simulink subsystem "frame_ctrl"  (R2021b)
settings: Solver=VariableStepAuto  StartTime=0.0  StopTime=10.0  RelTol=1e-3
undefined symbols (not defined in the file or in its folder): bank_bitwidth, fn_bitwidth, id_bitwidth
settings Model: Creator=torha  LastModifiedBy=torha
settings SolverCC: AlgebraicLoopSolver=TrustRegion
settings DebuggingCC: SFMachineParentedDataDiag=warning

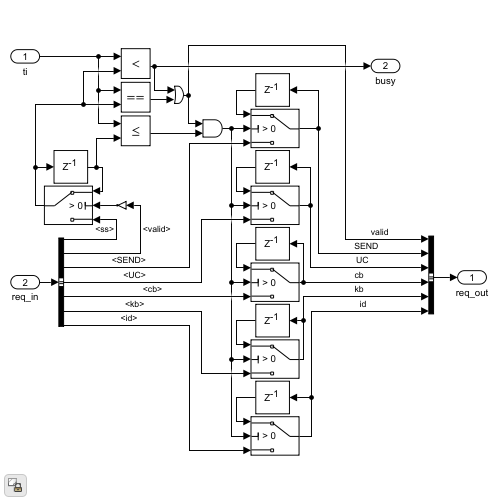
[thumbnail: Simulink's stored preview of the top-level diagram]
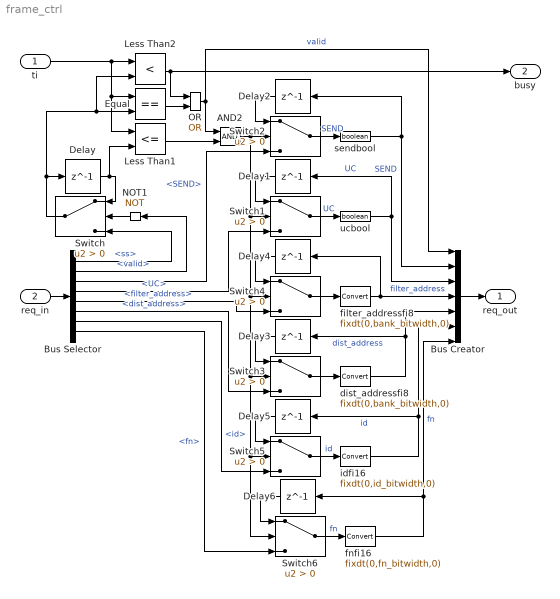
== system frame_ctrl ==
  ti : Inport
  req_in : Inport  Port=2
  AND2 : Logic  IconShape=distinctive  AllPortsSameDT=off  OutDataTypeStr=boolean
  Bus Creator : BusCreator  Inputs=7
  Bus Selector : BusSelector  OutputSignals=req.ss,valid,req.SEND,req.UC,req.filter_address,req.dist_address,id,req.fn
  Delay : Delay  DelayLength=1  InitialCondition=0
  Delay1 : Delay  DelayLength=1  InitialCondition=false
  Delay2 : Delay  DelayLength=1  InitialCondition=false
  Delay3 : Delay  DelayLength=1  InitialCondition=fi(0, false, bank_bitwidth, 0)
  Delay4 : Delay  DelayLength=1  InitialCondition=fi(0, false, bank_bitwidth, 0)
  Delay5 : Delay  DelayLength=1  InitialCondition=fi(0, false, id_bitwidth, 0)
  Delay6 : Delay  DelayLength=1  InitialCondition=fi(0, false, fn_bitwidth, 0)
  Equal : RelationalOperator  Operator===  OutDataTypeStr=boolean  RndMeth=Simplest
  Less Than1 : RelationalOperator  Operator=<=  OutDataTypeStr=boolean  RndMeth=Simplest
  Less Than2 : RelationalOperator  Operator=<  OutDataTypeStr=boolean  RndMeth=Simplest
  NOT1 : Logic  Operator=NOT  IconShape=distinctive  AllPortsSameDT=off  OutDataTypeStr=boolean
  OR : Logic  Operator=OR  IconShape=distinctive  AllPortsSameDT=off  OutDataTypeStr=boolean
  Switch{,1..6} (7 alike) : Switch  Criteria=u2 > Threshold
  dist_addressfi8 : DataTypeConversion  OutDataTypeStr=fixdt(0,bank_bitwidth,0)
  filter_addressfi8 : DataTypeConversion  OutDataTypeStr=fixdt(0,bank_bitwidth,0)
  fnfi16 : DataTypeConversion  OutDataTypeStr=fixdt(0,fn_bitwidth,0)
  idfi16 : DataTypeConversion  OutDataTypeStr=fixdt(0,id_bitwidth,0)
  sendbool : DataTypeConversion  OutDataTypeStr=boolean
  ucbool : DataTypeConversion  OutDataTypeStr=boolean
  req_out : Outport
  busy : Outport  Port=2
  wires:
  Switch6/1 -> fnfi16/1  "fn"
  Bus Selector/8 -> Switch6/3  "<fn>"
  fnfi16/1 -> Bus Creator/7, Delay6/1  "fn"
  Delay6/1 -> Switch6/1
  idfi16/1 -> Delay5/1, Bus Creator/6  "id"
  Switch3/1 -> dist_addressfi8/1
  Switch4/1 -> filter_addressfi8/1
  Switch1/1 -> ucbool/1  "UC"
  Switch2/1 -> sendbool/1  "SEND"
  Equal/1 -> OR/2
  Less Than2/1 -> OR/1, busy/1
  dist_addressfi8/1 -> Delay3/1, Bus Creator/5  "dist_address"
  filter_addressfi8/1 -> Delay4/1, Bus Creator/4  "filter_address"
  Bus Selector/7 -> Switch5/3  "<id>"
  Delay5/1 -> Switch5/1
  Switch5/1 -> idfi16/1  "id"
  Bus Selector/6 -> Switch3/3  "<dist_address>"
  Bus Selector/5 -> Switch4/3  "<filter_address>"
  Bus Selector/4 -> Switch1/3  "<UC>"
  Bus Selector/3 -> Switch2/3  "<SEND>"
  Delay4/1 -> Switch4/1
  AND2/1 -> Switch2/2, Switch6/2, Switch5/2, Switch3/2, Switch4/2, Switch1/2
  Delay3/1 -> Switch3/1
  Delay2/1 -> Switch2/1
  sendbool/1 -> Delay2/1, Bus Creator/2  "SEND"
  Less Than1/1 -> AND2/2
  ti/1 -> Equal/1, Less Than1/1, Less Than2/1
  Bus Selector/2 -> NOT1/1  "<valid>"
  NOT1/1 -> Switch/2
  ucbool/1 -> Bus Creator/3, Delay1/1  "UC"
  Delay1/1 -> Switch1/1
  Bus Selector/1 -> Switch/3  "<ss>"
  Switch/1 -> Equal/2, Less Than2/2, Delay/1
  Delay/1 -> Switch/1, Less Than1/2
  OR/1 -> Bus Creator/1, AND2/1  "valid"
  Bus Creator/1 -> req_out/1
  req_in/1 -> Bus Selector/1
